simulink model "FuzzyPID"  (R2015a)
settings: Solver=ode4  SolverMode=SingleTasking  StartTime=0.0  StopTime=inf  FixedStep=0.1  RelTol=1e-3
undefined symbols (not defined in the file or in its folder): Position
libraries: robotlib x8, fuzblock x1
settings Model: CovMetricSettings=dwe  CovHtmlReporting=off  covSaveCumulativeToWorkspaceVar=off  CovSaveSingleToWorkspaceVar=off  CovExternalEMLEnable=on  Creator=DwigHT  LastModifiedBy=DwigHT
settings DataIOCC: LimitDataPoints=off  SaveFormat=Dataset  ReturnWorkspaceOutputs=on
settings OptimizationCC: EnhancedBackFolding=on  PassReuseOutputArgsAs=Individual arguments  ZeroExternalMemoryAtStartup=off  ZeroInternalMemoryAtStartup=off  OptimizeModelRefInitCode=on  MaxStackSize=64
settings DebuggingCC: ParameterTunabilityLossMsg=error  UnconnectedInputMsg=none  UnconnectedOutputMsg=none  UnconnectedLineMsg=none  SFUnexpectedBacktrackingDiag=error  SFNoUnconditionalDefaultTransitionDiag=error
settings HardwareCC: ProdHWDeviceType=Generic->Unspecified (assume 32-bit Generic)
settings ModelReferenceCC: PropagateSignalLabelsOutOfModel=on
settings SFSimCC: SimUseLocalCustomCode=on
settings RTWCC: Description=Embedded Coder  SystemTargetFile=ert.tlc  TLCOptions="-aInlineSetEventsForThisBaseRateFcn=TLC_FALSE -aSuppressMultiTaskScheduler=TLC_FALSE  -aRateBasedStepFcn=0"  TemplateMakefile=ert_default_tmf  RTWUseLocalCustomCode=on  Toolchain=Catkin  TargetLang=C++
settings CodeAppCC: ForceParamTrailComments=on  IgnoreCustomStorageClasses=off  OperatorAnnotations=on  SimulinkDataObjDesc=on  SFDataObjDesc=on  InsertBlockDesc=on
settings ERTTargetCC: MultiwordLength=256  GenerateSampleERTMain=off  ParMdlRefBuildCompliant=on  CompOptLevelCompliant=on  ConcurrentExecutionCompliant=on  SupportContinuousTime=off  SupportVariableSizeSignals=off  ModelStepFunctionPrototypeControlCompliant=on  CPPClassGenCompliant=on  InlinedParameterPlacement=Hierarchical  ConvertIfToSwitch=on  SuppressUnreachableDefaultCases=on

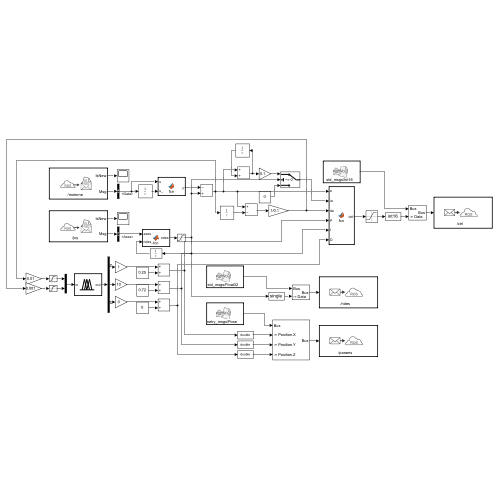
[thumbnail: Simulink's stored preview of the top-level diagram]
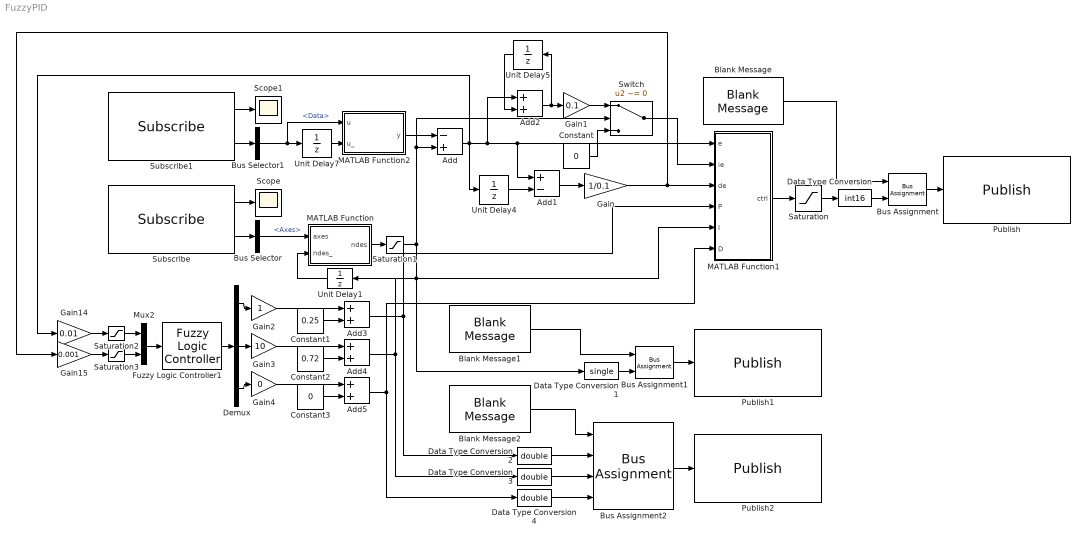
== system FuzzyPID ==
  Add : Sum  Inputs=-+
  Add1 : Sum  Inputs=+-
  Add{2..5} (4 alike) : Sum
  Blank Message : robotlib/Blank Message  messageClass=Message  entityType=std_msgs/Int16  messageType=std_msgs/Int16  SampleTime=inf  legacyBusStruct=off
  Blank Message1 : robotlib/Blank Message  messageClass=Message  entityType=std_msgs/Float32  messageType=std_msgs/Float32  SampleTime=inf  legacyBusStruct=off
  Blank Message2 : robotlib/Blank Message  messageClass=Message  entityType=geometry_msgs/Pose  messageType=geometry_msgs/Pose  SampleTime=inf  legacyBusStruct=off
  Bus Assignment : BusAssignment  AssignedSignals=Data
  Bus Assignment1 : BusAssignment  AssignedSignals=Data
  Bus Assignment2 : BusAssignment  AssignedSignals=Position.X,Position.Y,Position.Z
  Bus Selector : BusSelector  OutputSignals=Axes
  Bus Selector1 : BusSelector  OutputSignals=Data
  Constant : Constant  Value=0
  Constant1 : Constant  Value=0.25
  Constant2 : Constant  Value=0.72
  Constant3 : Constant  Value=0
  Data Type Conversion : DataTypeConversion  OutDataTypeStr=int16
  Data Type Conversion1 : DataTypeConversion  OutDataTypeStr=single
  Data Type Conversion2 : DataTypeConversion  OutDataTypeStr=double
  Data Type Conversion3 : DataTypeConversion  OutDataTypeStr=double
  Data Type Conversion4 : DataTypeConversion  OutDataTypeStr=double
  Demux : Demux  Outputs=3
  Fuzzy Logic Controller1 : fuzblock/Fuzzy Logic  Controller  FIS='fuzzpid.fis'
  Gain : Gain  Gain=1/0.1
  Gain1 : Gain  Gain=0.1
  Gain14 : Gain  Gain=0.01
  Gain15 : Gain  Gain=0.001
  Gain2 : Gain
  Gain3 : Gain  Gain=10
  Gain4 : Gain  Gain=0
  MATLAB Function : MATLAB Function  TreatAsAtomicUnit=on
      settings: PermitHierarchicalResolution=ParametersOnly
  MATLAB Function1 : MATLAB Function  TreatAsAtomicUnit=on
      settings: PermitHierarchicalResolution=ParametersOnly
  MATLAB Function2 : MATLAB Function  TreatAsAtomicUnit=on
      settings: PermitHierarchicalResolution=ParametersOnly
  Mux2 : Mux  Inputs=2
  Publish : robotlib/Publish  topicSource=Specify your own  topic=/ctrl  messageType=std_msgs/Int16  legacyBusStruct=off  messageQueueLength=1
  Publish1 : robotlib/Publish  topicSource=Specify your own  topic=/ndes  messageType=std_msgs/Float32  legacyBusStruct=off  messageQueueLength=1
  Publish2 : robotlib/Publish  topicSource=Specify your own  topic=/params  messageType=geometry_msgs/Pose  legacyBusStruct=off  messageQueueLength=1
  Saturation : Saturate  UpperLimit=255  LowerLimit=0
  Saturation1 : Saturate  UpperLimit=250  LowerLimit=0  OutDataTypeStr=double
  Saturation2 : Saturate  UpperLimit=3  LowerLimit=-3
  Saturation3 : Saturate  UpperLimit=3  LowerLimit=-3
  Scope : Scope
      settings: TimeRange=auto  MaxDataPoints=5000  SaveToWorkspace=off  SaveName=ScopeData  YMin=-10  YMax=10  SampleTime=-1
  Scope1 : Scope
      settings: TimeRange=auto  MaxDataPoints=5000  SaveToWorkspace=off  YMin=-10  YMax=10  SampleTime=-1
  Subscribe : robotlib/Subscribe  topicSource=Select from ROS network  topic=/joy  messageType=sensor_msgs/Joy  SampleTime=-1  legacyBusStruct=off  messageQueueLength=1
  Subscribe1 : robotlib/Subscribe  topicSource=Specify your own  topic=/motorne  messageType=std_msgs/Float32  SampleTime=-1  legacyBusStruct=off  messageQueueLength=1
  Switch : Switch  Criteria=u2 ~= 0
  Unit Delay{1,4..5,7} (4 alike) : UnitDelay  SampleTime=-1  HasFrameUpgradeWarning=on
  wires:
  Subscribe/2 -> Bus Selector/1
  Subscribe/1 -> Scope/1
  Bus Assignment/1 -> Publish/1
  Blank Message/1 -> Bus Assignment/1
  Bus Selector/1 -> MATLAB Function/1(axes)  "<Axes>"
  Data Type Conversion/1 -> Bus Assignment/2
  Saturation/1 -> Data Type Conversion/1
  MATLAB Function/1(ndes) -> Saturation1/1
  Add5/1 -> Data Type Conversion4/1, MATLAB Function1/6(D)
  Add4/1 -> Data Type Conversion3/1, MATLAB Function1/5(I)
  Add3/1 -> Data Type Conversion2/1, MATLAB Function1/4(P)
  Subscribe1/1 -> Scope1/1
  Subscribe1/2 -> Bus Selector1/1
  Bus Selector1/1 -> MATLAB Function2/1(u), Unit Delay7/1  "<Data>"
  Unit Delay4/1 -> Add1/2
  Add/1 -> Unit Delay4/1, Gain14/1, MATLAB Function1/1(e), Add1/1, Add2/1
  Add1/1 -> Gain/1
  Gain/1 -> Gain15/1, MATLAB Function1/3(de)
  Add2/1 -> Gain1/1, Unit Delay5/1
  Unit Delay5/1 -> Add2/2
  MATLAB Function1/1(ctrl) -> Saturation/1
  Bus Assignment1/1 -> Publish1/1
  Blank Message1/1 -> Bus Assignment1/1
  Data Type Conversion1/1 -> Bus Assignment1/2
  Blank Message2/1 -> Bus Assignment2/1
  Bus Assignment2/1 -> Publish2/1
  MATLAB Function2/1(y) -> Add/1
  Unit Delay7/1 -> MATLAB Function2/2(u_)
  Data Type Conversion2/1 -> Bus Assignment2/2
  Data Type Conversion3/1 -> Bus Assignment2/3
  Data Type Conversion4/1 -> Bus Assignment2/4
  Gain1/1 -> Switch/1
  Switch/1 -> MATLAB Function1/2(ie)
  Constant/1 -> Switch/3
  Fuzzy Logic Controller1/1 -> Demux/1
  Demux/1 -> Gain2/1
  Demux/2 -> Gain3/1
  Demux/3 -> Gain4/1
  Gain2/1 -> Add3/1
  Gain3/1 -> Add4/1
  Gain4/1 -> Add5/1
  Constant1/1 -> Add3/2
  Constant2/1 -> Add4/2
  Constant3/1 -> Add5/2
  Mux2/1 -> Fuzzy Logic Controller1/1
  Saturation2/1 -> Mux2/1
  Saturation3/1 -> Mux2/2
  Gain15/1 -> Saturation3/1
  Gain14/1 -> Saturation2/1
  Saturation1/1 -> Unit Delay1/1, Data Type Conversion1/1, Switch/2, Add/2
  Unit Delay1/1 -> MATLAB Function/2(ndes_)

== matlab function FuzzyPID/MATLAB Function1 ==
  data: e input; ctrl output; ie input; de input; P input; I input; D input
function ctrl = fcn(e,ie,de,P,I,D)

ctrl = P*e+I*ie+D*de;

== matlab function FuzzyPID/MATLAB Function ==
  data: axes input; ndes output; ndes_ input
function ndes = fcn(axes,ndes_)
    ndes = ndes_+axes(8)*50;
end

== matlab function FuzzyPID/MATLAB Function2 ==
  data: u input; y output; u_ input
function y = fcn(u, u_)
if u<0
    y = u_;
else
    y = u;
end
